simulink library "lib_OBC_Manager"  (R2017a)
settings: Solver=VariableStepAuto  StartTime=0.0  StopTime=10.0  RelTol=1e-3
libraries: simulink x7, powerlib_meascontrol x1
settings Model: Creator=Vraj M  LastModifiedBy=Vraj M

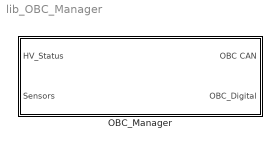
== system lib_OBC_Manager ==
  OBC_Manager : Subsystem

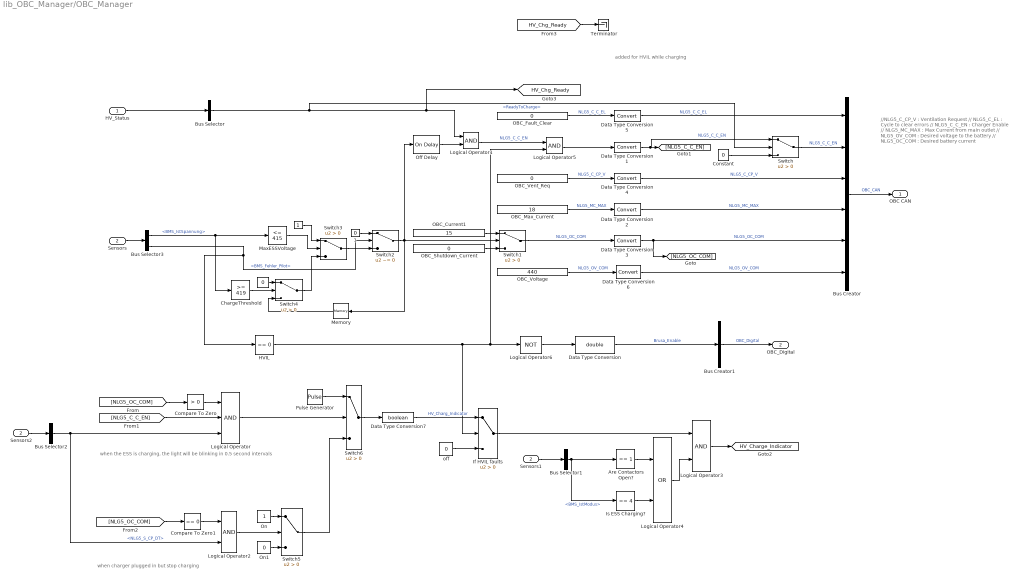
== system lib_OBC_Manager/OBC_Manager ==
  note: added for HVIL
      | while charging
  note: //NLG5_C_CP_V : Ventilation Request
      | // NLG5_C_EL : Cycle to clear errors
      | // NLG5_C_C_EN : Charger Enable
      | // NLG5_MC_MAX : Max Current from main outlet
      | // NLG5_OV_COM : Desired voltage to the battery
      | // NLG5_OC_COM : Desired battery current
  note: when charger plugged in but stop charging
  note: when the ESS is charging, the light will be blinking in 0.5 second intervals
  HV_Status : Inport
  Sensors : Inport  Port=2
  " " : Constant
  "   " : Constant  Value=0
  "   1" : Constant  Value=0
  Are Contactors Open? : simulink/Logic and Bit Operations/Compare To Constant  relop===  const=1  OutDataTypeStr=boolean
  Bus Creator : BusCreator  Inputs=6
  Bus Creator1 : BusCreator  Inputs=1
  Bus Selector : BusSelector  OutputSignals=ReadyToCharge
  Bus Selector1 : BusSelector  OutputSignals=from_CAN.fromHV_CAN.from_BMSHybrid.BMS_HYB_02.BMS_IstModus
  Bus Selector2 : BusSelector  OutputSignals=from_CAN.fromHV_CAN.from_OBC.NLG5_ST.NLG5_S_CP_DT
  Bus Selector3 : BusSelector  OutputSignals=from_CAN.fromHV_CAN.from_BMSHybrid.BMS_HYB_02.BMS_IstSpannung,from_CAN.fromHV_CAN.from_BMSHybrid.BMS_HYB_02.BMS_Fehler_Pilot
  ChargeThreshold : simulink/Logic and Bit Operations/Compare To Constant  relop=>=  const=419  OutDataTypeStr=boolean
  Compare To Zero : simulink/Logic and Bit Operations/Compare To Zero  relop=>  OutDataTypeStr=boolean
  Compare To Zero1 : simulink/Logic and Bit Operations/Compare To Zero  relop===  OutDataTypeStr=boolean
  Constant : Constant  Value=0
  Data Type Conversion : DataTypeConversion  OutDataTypeStr=double
  Data Type Conversion{1..6} (6 alike) : DataTypeConversion
  Data Type Conversion7 : DataTypeConversion  OutDataTypeStr=boolean
  HVIL : simulink/Logic and Bit Operations/Compare To Constant  relop===  const=0  OutDataTypeStr=boolean
  If HVIL faults : Switch  Criteria=u2 > Threshold
  Is ESS Charging? : simulink/Logic and Bit Operations/Compare To Constant  relop===  const=4  OutDataTypeStr=boolean
  Logical Operator : Logic  Inputs=3  AllPortsSameDT=off  OutDataTypeStr=boolean
  Logical Operator{1..3,5} (4 alike) : Logic  AllPortsSameDT=off  OutDataTypeStr=boolean
  Logical Operator4 : Logic  Operator=OR  AllPortsSameDT=off  OutDataTypeStr=boolean
  Logical Operator6 : Logic  Operator=NOT  Inputs=3  AllPortsSameDT=off  OutDataTypeStr=boolean
  MaxESSVoltage : simulink/Logic and Bit Operations/Compare To Constant  relop=<=  const=415  OutDataTypeStr=boolean
  Memory : Memory  InheritSampleTime=on
  OBC_Current1 : Constant  Value=15
  OBC_Fault_Clear : Constant  Value=0
  OBC_Max_Current : Constant  Value=18
  OBC_Shutdown_Current : Constant  Value=0
  OBC_Vent_Req : Constant  Value=0
  OBC_Voltage : Constant  Value=440
  Off Delay : powerlib_meascontrol/Logic/On Delay  DelayType=Off delay  delay=30  ic=0  Ts=0
      settings: SourceProductName=Simscape Power Systems
  On : Constant
  On1 : Constant  Value=0
  Pulse Generator : DiscretePulseGenerator  PulseType=Time based  Period=1  PulseWidth=50
  Sensors1 : InportShadow  Port=2
  Sensors2 : InportShadow  Port=2
  Switch{,1,3..6} (6 alike) : Switch  Criteria=u2 > Threshold
  Switch2 : Switch  Criteria=u2 ~= 0
  Terminator : Terminator
  off : Constant  Value=0
  OBC CAN : Outport
  OBC_Digital : Outport  Port=2
  tag scope: HV_Charge_Indicator=global, HV_Chg_Ready=global
  wires:
  Data Type Conversion7/1 -> If HVIL faults/1  "HV_Charg_Indicator"
  OBC_Voltage/1 -> Data Type Conversion6/1  "NLG5_OV_COM"
  OBC_Max_Current/1 -> Data Type Conversion2/1  "NLG5_MC_MAX"
  OBC_Fault_Clear/1 -> Data Type Conversion5/1  "NLG5_C_C_EL"
  OBC_Vent_Req/1 -> Data Type Conversion4/1  "NLG5_C_CP_V"
  Switch1/1 -> Data Type Conversion3/1  "NLG5_OC_COM"
  Logical Operator1/1 -> Logical Operator5/1  "NLG5_C_C_EN"
  Data Type Conversion1/1 -> Switch/1, [NLG5_C_C_EN]  "NLG5_C_C_EN"
  Switch4/1 -> Switch3/3
  Memory/1 -> Switch4/3
  OBC_Shutdown_Current/1 -> Switch1/3
  " "/1 -> Switch3/1
  ChargeThreshold/1 -> Switch4/2
  "   "/1 -> Switch4/1
  Switch2/1 -> Memory/1, Off Delay/1, Switch1/2
  OBC_Current1/1 -> Switch1/1
  Data Type Conversion3/1 -> Bus Creator/5, [NLG5_OC_COM]  "NLG5_OC_COM"
  Data Type Conversion6/1 -> Bus Creator/6  "NLG5_OV_COM"
  Data Type Conversion4/1 -> Bus Creator/3  "NLG5_C_CP_V"
  Data Type Conversion5/1 -> Bus Creator/1  "NLG5_C_C_EL"
  Data Type Conversion2/1 -> Bus Creator/4  "NLG5_MC_MAX"
  Bus Selector3/1 -> ChargeThreshold/1, MaxESSVoltage/1  "<BMS_IstSpannung>"
  Off Delay/1 -> Logical Operator1/2
  Bus Selector/1 -> Switch/2, Logical Operator1/1, [HV_Chg_Ready]  "<ReadyToCharge>"
  MaxESSVoltage/1 -> Switch3/2
  HV_Status/1 -> Bus Selector/1
  Bus Creator/1 -> OBC CAN/1  "OBC_CAN"
  Sensors/1 -> Bus Selector3/1
  [NLG5_OC_COM] -> Compare To Zero/1
  Compare To Zero/1 -> Logical Operator/1
  [NLG5_C_C_EN] -> Logical Operator/2
  Logical Operator/1 -> Switch6/2
  Pulse Generator/1 -> Switch6/1
  [NLG5_OC_COM] -> Compare To Zero1/1
  Compare To Zero1/1 -> Logical Operator2/1
  Logical Operator2/1 -> Switch5/2
  On/1 -> Switch5/1
  On1/1 -> Switch5/3
  Switch5/1 -> Switch6/3
  Switch6/1 -> Data Type Conversion7/1
  Bus Selector3/2 -> HVIL/1, Switch2/2  "<BMS_Fehler_Pilot>"
  Data Type Conversion/1 -> Bus Creator1/1  "Brusa_Enable"
  Bus Creator1/1 -> OBC_Digital/1  "OBC_Digital"
  Switch3/1 -> Switch2/3
  "   1"/1 -> Switch2/1
  HVIL/1 -> Logical Operator5/2, Logical Operator6/1, If HVIL faults/2
  If HVIL faults/1 -> Logical Operator3/1
  off/1 -> If HVIL faults/3
  Logical Operator3/1 -> [HV_Charge_Indicator]
  Sensors1/1 -> Bus Selector1/1
  Are Contactors Open?/1 -> Logical Operator4/1
  Bus Selector1/1 -> Is ESS Charging?/1, Are Contactors Open?/1  "<BMS_IstModus>"
  Is ESS Charging?/1 -> Logical Operator4/2
  Logical Operator4/1 -> Logical Operator3/2
  Logical Operator5/1 -> Data Type Conversion1/1
  Logical Operator6/1 -> Data Type Conversion/1
  Constant/1 -> Switch/3
  Switch/1 -> Bus Creator/2  "NLG5_C_C_EN"
  Sensors2/1 -> Bus Selector2/1
  Bus Selector2/1 -> Logical Operator2/2, Logical Operator/3  "<NLG5_S_CP_DT>"
  [HV_Chg_Ready] -> Terminator/1
